simulink model "sampleModel2120_pp_difftest"  (R2021a)
settings: Solver=VariableStepAuto  StartTime=0.0  StopTime=10.0  RelTol=1e-3
undefined symbols (not defined in the file or in its folder): DiscIntNeverNeededParam, magnitude, Newton, Raphson
libraries: simulink x67, pid_lib x12
(part 1 of 3)
settings Model: Creator=lenovo  LastModifiedBy=user

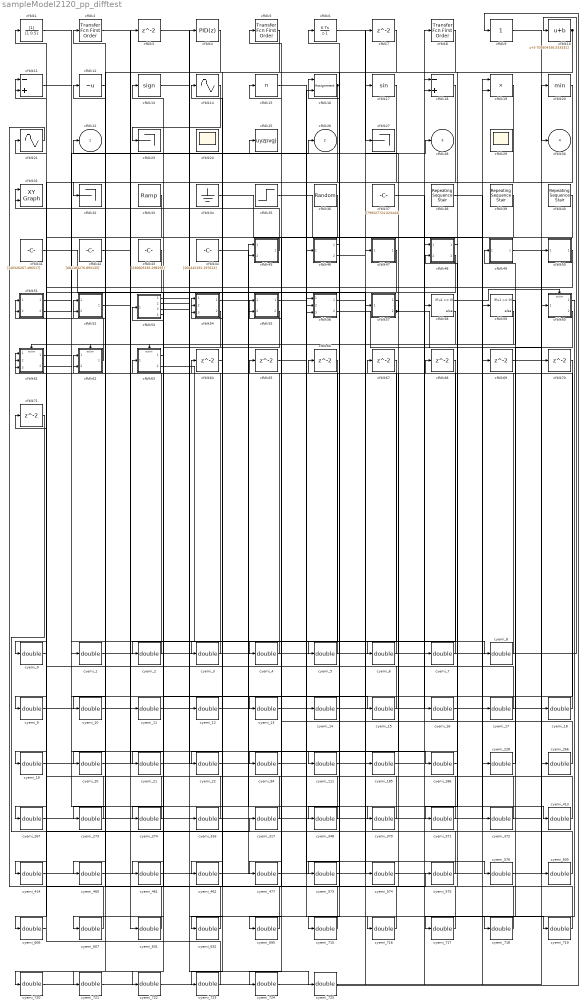
== system sampleModel2120_pp_difftest ==
  cfblk1 : DiscreteFilter  SampleTime=1
  cfblk10 : Bias  Bias=[-709504336.533331]
  cfblk11 : Sum  Inputs=-+  OutDataTypeStr=double
  cfblk12 : UnaryMinus
  cfblk13 : Signum
  cfblk14 : Sin  TimeSource=Use external signal  SampleTime=0
  cfblk15 : Product  Inputs=*  OutDataTypeStr=double
  cfblk16 : Assignment  DiagnosticForDimensions=Warning  IndexOptions=Index vector (dialog)  Indices=1  OutputSizes=1
  cfblk17 : Trigonometry
  cfblk18 : Sum  Inputs=-+  OutDataTypeStr=double
  cfblk19 : Product  Inputs=**  OutDataTypeStr=double
  cfblk2 : simulink/Discrete/Transfer Fcn First Order  PoleZ=0.95  ICPrevOutput=0.0  DoSatur=off
  cfblk20 : MinMax  OutDataTypeStr=double
  cfblk21 : Sin  TimeSource=Use external signal  SampleTime=0
  cfblk23 : Terminator
  cfblk24 : Scope
      settings: Floating=on
  cfblk25 : ToWorkspace  VariableName=uyzpvgj  SaveFormat=Timeseries  SampleTime=-1
  cfblk27 : Terminator
  cfblk29 : Scope
      settings: Floating=on
  cfblk{3,7,64..71} (10 alike) : Delay  SampleTime=1
  cfblk31 : simulink/Sinks/XY Graph  xmin=-1  xmax=1  ymin=-1  ymax=1  st=-1
  cfblk32 : Terminator
  cfblk33 : simulink/Sources/Ramp  slope=[-9170.423728]  start=[47.124759]  InitialOutput=[-914026.200250]
  cfblk34 : Ground
  cfblk35 : Step  Time=[9.000000]  Before=[-795213372.799819]  After=[478961987.281532]  SampleTime=0
  cfblk36 : RandomNumber  Mean=[10617.420643]  Variance=[21176.794349]  Seed=[230646429.000000]  SampleTime=0.1
  cfblk37 : Constant  Value=[799327724.023444]  OutDataTypeStr=double  SampleTime=1
  cfblk38 : simulink/Sources/Repeating Sequence Stair  OutValues=[-433408772.823916, -415254257.712957]  tsamp=1  OutMin=[]  OutMax=[]  OutDataTypeStr=double  OutputDataTypeScalingMode=double  OutDataType=fixdt(0,8)  ConRadixGroup=Best Precision: Vector-wise  OutScaling=2^-12
  cfblk39 : simulink/Sources/Repeating Sequence Stair  OutValues=[-289850517.751217, -807875800.203243]  tsamp=1  OutMin=[]  OutMax=[]  OutDataTypeStr=double  OutputDataTypeScalingMode=double  OutDataType=fixdt(0,8)  ConRadixGroup=Best Precision: Vector-wise  OutScaling=2^-12
  cfblk4 : pid_lib/PID Controller  Controller=PID  Form=Parallel  TimeDomain=Discrete-time  UseExternalTs=off  SampleTime=1  IntegratorMethod=Forward Euler  FilterMethod=Forward Euler  ControllerParametersSource=internal  P=1  I=1  D=0  UseFilter=on  N=100  TunerSelectOption=Transfer Function Based (PID Tuner App)  InitialConditionSource=internal  InitialConditionForIntegrator=0  InitialConditionForFilter=0  DifferentiatorICPrevScaledInput=0  ExternalReset=none  TrackingMode=off  Kt=1  LimitOutput=off  SatLimitsSource=internal  UpperSaturationLimit=inf  LowerSaturationLimit=-inf  LinearizeAsGain=off  AntiWindupMode=none  Kb=1  POutMin=[]  POutMax=[]  IOutMin=[]  IOutMax=[]  DOutMin=[]  DOutMax=[]  NOutMin=[]  NOutMax=[]  SumOutMin=[]  SumOutMax=[]  SaturationOutMin=[]  SaturationOutMax=[]  PParamMin=[]  PParamMax=[]  IParamMin=[]  IParamMax=[]  DParamMin=[]  DParamMax=[]  NParamMin=[]  NParamMax=[]  KbParamMin=[]  KbParamMax=[]  KtParamMin=[]  KtParamMax=[]  KbOutMin=[]  KbOutMax=[]  KtOutMin=[]  KtOutMax=[]  IntegratorOutMin=[]  IntegratorOutMax=[]  FilterOutMin=[]  FilterOutMax=[]  SumI1OutMin=[]  SumI1OutMax=[]  SumI2OutMin=[]  SumI2OutMax=[]  SumI3OutMin=[]  SumI3OutMax=[]  SumI4OutMin=[]  SumI4OutMax=[]  SumDOutMin=[]  SumDOutMax=[]  DifferentiatorOutMin=[]  DifferentiatorOutMax=[]  FilterDiffOutCoefMin=[]  FilterDiffOutCoefMax=[]  ReciprocalOutMin=[]  ReciprocalOutMax=[]  SumDenOutMin=[]  SumDenOutMax=[]  SumNumOutMin=[]  SumNumOutMax=[]  DivideOutMin=[]  DivideOutMax=[]  UdiffTsProdOutMin=[]  UdiffTsProdOutMax=[]  NTsProdOutMin=[]  NTsProdOutMax=[]  UintegralTsProdOutMin=[]  UintegralTsProdOutMax=[]  UngainTsProdOutMin=[]  UngainTsProdOutMax=[]  IntegratorContinuousStateAttributes=''  IntegratorStateMustResolveToSignalObject=off  IntegratorRTWStateStorageClass=Auto  FilterContinuousStateAttributes=''  FilterStateMustResolveToSignalObject=off  FilterRTWStateStorageClass=Auto  ParallelPVariant=InternalParameters  IdealPVariant=Disabled  IVariant=InternalParameters  DVariant=InternalParameters  IntegratorVariant=Discrete  SatVariant=Disabled  AWVariant=Passthrough  PCopyVariant=Disabled  TRVariant=Disabled  FdbkBlocksVariant=Forward  IdealPFdbkVariant=Disabled  SatFdbkVariant=Disabled  DerivativeFilterVariant=ForwardEulerFilter  NVariant=InternalParameters  NCopyVariant=Disabled  FilterICVariant=InternalICsFilter  IntegratorICVariant=InternalICs  ExternalResetVariant=Disabled  TRSumVariant=Passthrough  SumFdbkVariant=Disabled  SumVariant=Sum_PID  TsampFilterVariant=InternalTs  TsampNgainVariant=Passthrough  TsampIntegralVariant=Passthrough  ExternalSaturationOutDataTypeStr=Inherit: Same as second input
  cfblk40 : simulink/Sources/Repeating Sequence Stair  OutValues=[599228246.238422, -891664695.317547]  tsamp=1  OutMin=[]  OutMax=[]  OutDataTypeStr=double  OutputDataTypeScalingMode=double  OutDataType=fixdt(0,8)  ConRadixGroup=Best Precision: Vector-wise  OutScaling=2^-12
  cfblk41 : Constant  Value=[140326207.496517]  OutDataTypeStr=double  SampleTime=1
  cfblk42 : Constant  Value=[681184276.893135]  OutDataTypeStr=double  SampleTime=1
  cfblk43 : Constant  Value=[230605335.298195]  OutDataTypeStr=double  SampleTime=1
  cfblk44 : Constant  Value=[206442191.197613]  OutDataTypeStr=double  SampleTime=1
  cfblk45 : Subsystem
  cfblk46 : Subsystem
  cfblk47 : Subsystem
  cfblk48 : Subsystem
  cfblk49 : Subsystem
  cfblk5 : simulink/Discrete/Transfer Fcn First Order  PoleZ=0.95  ICPrevOutput=0.0  DoSatur=off
  cfblk50 : Subsystem
  cfblk51 : Subsystem
  cfblk52 : Subsystem
  cfblk53 : Subsystem
  cfblk54 : Subsystem
  cfblk55 : Subsystem
  cfblk56 : Subsystem
  cfblk57 : Subsystem
  cfblk58 : If  IfExpression=u1 >= 0  SampleTime=1
  cfblk59 : If  IfExpression=u1 >= 0  SampleTime=1
  cfblk6 : DiscreteIntegrator  OutDataTypeStr=double  ICPrevOutput=DiscIntNeverNeededParam  ICPrevScaledInput=DiscIntNeverNeededParam
  cfblk60 : Subsystem  TreatAsAtomicUnit=on
  cfblk61 : Subsystem  TreatAsAtomicUnit=on
  cfblk62 : Subsystem  TreatAsAtomicUnit=on
  cfblk63 : Subsystem  TreatAsAtomicUnit=on
  cfblk8 : simulink/Discrete/Transfer Fcn First Order  PoleZ=0.95  ICPrevOutput=0.0  DoSatur=off
  cfblk9 : simulink/Math Operations/Slider Gain  gain=1  low=0  high=2
  cyemi_{0..22,84,111,185..186,228,266..267,273..274,316..317,348,370..372,413..414,460..462,477,573..576,605..607,631..632,695,715..725} (65 alike) : DataTypeConversion  OutDataTypeStr=double
  cfblk22 : Outport
  cfblk26 : Outport  Port=2
  cfblk28 : Outport  Port=3
  cfblk30 : Outport  Port=4
  wires:
  cfblk45/1(cfblk2) -> cfblk31/1
  cfblk9/1 -> cfblk30/1
  cfblk14/1 -> cfblk23/1
  cfblk51/2(cfblk12) -> cfblk26/1
  cfblk57/2(cfblk17) -> cfblk22/1, cyemi_372/1
  cfblk46/2(cfblk8) -> cfblk28/1
  cfblk62/1(cfblk2) -> cfblk31/2
  cfblk16/1 -> cyemi_22/1, cyemi_723/1
  cfblk6/1 -> cfblk27/1
  cfblk4/1 -> cfblk32/1
  cfblk10/1 -> cyemi_3/1, cyemi_371/1
  cfblk58/1 -> cfblk60/Action
  cfblk58/2 -> cfblk61/Action
  cfblk59/1 -> cfblk62/Action
  cfblk59/2 -> cfblk63/Action
  cyemi_0/1 -> cfblk1/1
  cfblk33/1 -> cyemi_0/1
  cyemi_1/1 -> cfblk10/1
  cfblk61/2(cfblk14) -> cyemi_1/1
  cyemi_2/1 -> cfblk11/1
  cfblk66/1 -> cyemi_2/1
  cyemi_3/1 -> cfblk11/2
  cyemi_4/1 -> cfblk12/1
  cfblk63/2(cfblk8) -> cyemi_4/1
  cyemi_5/1 -> cfblk13/1
  cfblk54/1(cfblk2) -> cyemi_5/1
  cyemi_6/1 -> cfblk14/1
  cfblk1/1 -> cyemi_6/1
  cyemi_7/1 -> cfblk15/1
  cfblk37/1 -> cyemi_7/1
  cyemi_8/1 -> cfblk16/1
  cfblk52/1(cfblk2) -> cyemi_8/1
  cyemi_9/1 -> cfblk16/2
  cfblk17/1 -> cyemi_9/1
  cyemi_10/1 -> cfblk17/1
  cfblk12/1 -> cyemi_10/1
  cyemi_11/1 -> cfblk18/1
  cfblk2/1 -> cyemi_11/1
  cyemi_12/1 -> cfblk18/2
  cfblk53/3(cfblk6) -> cyemi_12/1
  cyemi_13/1 -> cfblk19/1
  cfblk61/1(cfblk2) -> cyemi_13/1
  cyemi_14/1 -> cfblk19/2
  cfblk15/1 -> cyemi_14/1
  cyemi_15/1 -> cfblk2/1
  cfblk53/1(cfblk2) -> cyemi_15/1
  cyemi_16/1 -> cfblk20/1
  cfblk34/1 -> cyemi_16/1
  cyemi_17/1 -> cfblk21/1
  cfblk35/1 -> cyemi_17/1
  cyemi_18/1 -> cfblk25/1
  cfblk56/2(cfblk12) -> cyemi_18/1
  cyemi_19/1 -> cfblk3/1
  cfblk50/1(cfblk2) -> cyemi_19/1
  cyemi_20/1 -> cfblk4/1
  cfblk47/1(cfblk2) -> cyemi_20/1
  cyemi_21/1 -> cfblk45/1(cfblk1)
  cfblk54/2(cfblk12) -> cyemi_21/1
  cyemi_22/1 -> cfblk45/2(cfblk15)
  cyemi_84/1 -> cfblk46/1(cfblk1)
  cfblk48/1(cfblk2) -> cyemi_84/1
  cyemi_111/1 -> cfblk47/1(cfblk1)
  cfblk57/1(cfblk2) -> cyemi_111/1
  cyemi_185/1 -> cfblk48/1(cfblk1)
  cfblk41/1 -> cyemi_185/1
  cyemi_186/1 -> cfblk48/2(cfblk13)
  cfblk11/1 -> cyemi_186/1
  cyemi_228/1 -> cfblk49/1(cfblk1)
  cfblk38/1 -> cyemi_228/1
  cyemi_266/1 -> cfblk5/1
  cfblk69/1 -> cyemi_266/1
  cyemi_267/1 -> cfblk50/1(cfblk1)
  cfblk18/1 -> cyemi_267/1
  cyemi_273/1 -> cfblk51/1(cfblk1)
  cfblk8/1 -> cyemi_273/1
  cyemi_274/1 -> cfblk51/2(cfblk11)
  cfblk53/4(cfblk7) -> cyemi_274/1
  cyemi_316/1 -> cfblk52/1(cfblk1)
  cfblk13/1 -> cyemi_316/1
  cyemi_317/1 -> cfblk52/2(cfblk15)
  cfblk71/1 -> cyemi_317/1
  cyemi_348/1 -> cfblk53/1(cfblk1)
  cfblk46/1(cfblk2) -> cyemi_348/1
  cyemi_370/1 -> cfblk54/1(cfblk1)
  cfblk44/1 -> cyemi_370/1
  cyemi_371/1 -> cfblk54/2(cfblk10)
  cyemi_372/1 -> cfblk54/3(cfblk11)
  cyemi_413/1 -> cfblk55/1(cfblk1)
  cfblk51/1(cfblk2) -> cyemi_413/1
  cyemi_414/1 -> cfblk55/2(cfblk10)
  cfblk20/1 -> cyemi_414/1
  cyemi_460/1 -> cfblk56/1(cfblk1)
  cfblk5/1 -> cyemi_460/1
  cyemi_461/1 -> cfblk56/2(cfblk10)
  cfblk70/1 -> cyemi_461/1
  cyemi_462/1 -> cfblk56/3(cfblk11)
  cfblk64/1 -> cyemi_462/1
  cyemi_477/1 -> cfblk57/1(cfblk1)
  cfblk39/1 -> cyemi_477/1
  cyemi_573/1 -> cfblk58/1
  cfblk7/1 -> cyemi_573/1
  cyemi_574/1 -> cfblk59/1
  cfblk56/1(cfblk2) -> cyemi_574/1
  cyemi_575/1 -> cfblk6/1
  cfblk21/1 -> cyemi_575/1
  cyemi_576/1 -> cfblk60/1(cfblk1)
  cfblk65/1 -> cyemi_576/1
  cyemi_605/1 -> cfblk61/1(cfblk1)
  cfblk49/1(cfblk2) -> cyemi_605/1
  cyemi_606/1 -> cfblk61/2(cfblk12)
  cfblk43/1 -> cyemi_606/1
  cyemi_607/1 -> cfblk61/3(cfblk13)
  cfblk63/1(cfblk2) -> cyemi_607/1
  cyemi_631/1 -> cfblk62/1(cfblk1)
  cfblk42/1 -> cyemi_631/1
  cyemi_632/1 -> cfblk62/2(cfblk13)
  cfblk67/1 -> cyemi_632/1
  cyemi_695/1 -> cfblk63/1(cfblk1)
  cfblk68/1 -> cyemi_695/1
  cyemi_715/1 -> cfblk64/1
  cfblk19/1 -> cyemi_715/1
  cyemi_716/1 -> cfblk65/1
  cfblk53/2(cfblk5) -> cyemi_716/1
  cyemi_717/1 -> cfblk66/1
  cfblk60/1(cfblk2) -> cyemi_717/1
  cyemi_718/1 -> cfblk67/1
  cfblk60/2(cfblk14) -> cyemi_718/1
  cyemi_719/1 -> cfblk68/1
  cfblk55/1(cfblk2) -> cyemi_719/1
  cyemi_720/1 -> cfblk69/1
  cfblk55/2(cfblk11) -> cyemi_720/1
  cyemi_721/1 -> cfblk7/1
  cfblk40/1 -> cyemi_721/1
  cyemi_722/1 -> cfblk70/1
  cfblk48/2(cfblk14) -> cyemi_722/1
  cyemi_723/1 -> cfblk71/1
  cyemi_724/1 -> cfblk8/1
  cfblk36/1 -> cyemi_724/1
  cyemi_725/1 -> cfblk9/1
  cfblk3/1 -> cyemi_725/1

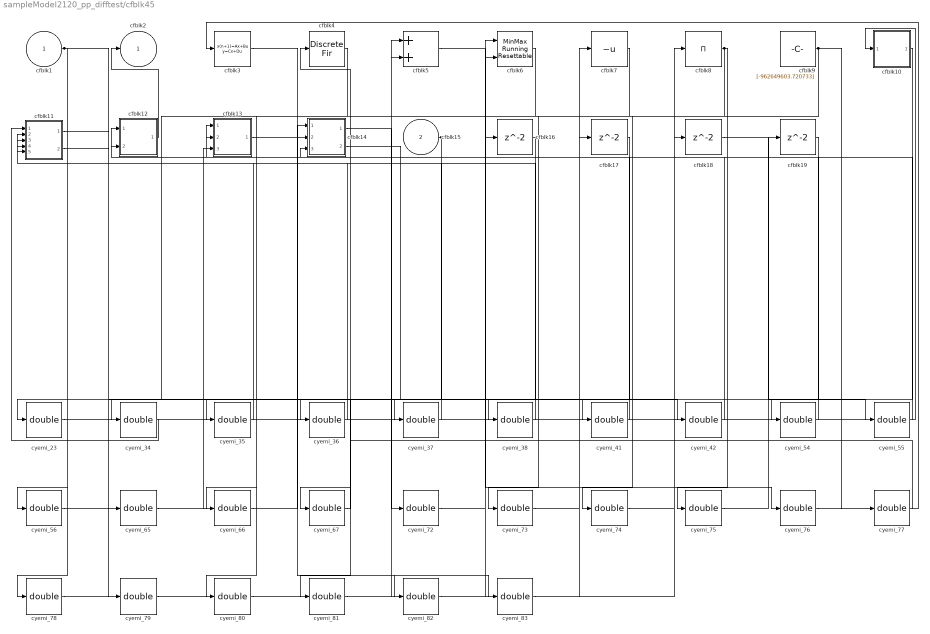
== system sampleModel2120_pp_difftest/cfblk45 ==
  cfblk1 : Inport
  cfblk15 : Inport  Port=2
  cfblk10 : Subsystem
  cfblk11 : Subsystem
  cfblk12 : Subsystem
  cfblk13 : Subsystem
  cfblk14 : Subsystem
  cfblk{16..19} (4 alike) : Delay  SampleTime=1
  cfblk3 : DiscreteStateSpace
  cfblk4 : DiscreteFir  SampleTime=1
  cfblk5 : Sum  OutDataTypeStr=double
  cfblk6 : simulink/Math Operations/MinMax Running Resettable  Function=min  vinit=0.0
  cfblk7 : UnaryMinus
  cfblk8 : Product  Inputs=*  OutDataTypeStr=double
  cfblk9 : Constant  Value=[-962649603.720733]  OutDataTypeStr=double  SampleTime=1
  cyemi_{23,34..38,41..42,54..56,65..67,72..83} (26 alike) : DataTypeConversion  OutDataTypeStr=double
  cfblk2 : Outport
  wires:
  cfblk12/1(cfblk2) -> cfblk2/1
  cfblk1/1 -> cyemi_23/1, cyemi_36/1, cyemi_42/1, cyemi_56/1
  cfblk9/1 -> cyemi_38/1, cyemi_77/1
  cfblk8/1 -> cyemi_73/1, cyemi_74/1, cyemi_75/1
  cyemi_23/1 -> cfblk10/1(cfblk1)
  cyemi_34/1 -> cfblk11/1(cfblk1)
  cfblk4/1 -> cyemi_34/1
  cyemi_35/1 -> cfblk11/2(cfblk6)
  cfblk6/1 -> cyemi_35/1
  cyemi_36/1 -> cfblk11/3(cfblk7)
  cyemi_37/1 -> cfblk11/4(cfblk8)
  cfblk19/1 -> cyemi_37/1
  cyemi_38/1 -> cfblk11/5(cfblk9)
  cyemi_41/1 -> cfblk12/1(cfblk1)
  cfblk14/2(cfblk9) -> cyemi_41/1
  cyemi_42/1 -> cfblk12/2(cfblk11)
  cyemi_54/1 -> cfblk13/1(cfblk1)
  cfblk10/1(cfblk2) -> cyemi_54/1
  cyemi_55/1 -> cfblk13/2(cfblk11)
  cfblk18/1 -> cyemi_55/1
  cyemi_56/1 -> cfblk13/3(cfblk12)
  cyemi_65/1 -> cfblk14/1(cfblk1)
  cfblk11/1(cfblk2) -> cyemi_65/1
  cyemi_66/1 -> cfblk14/2(cfblk7)
  cfblk15/1 -> cyemi_66/1, cyemi_67/1
  cyemi_67/1 -> cfblk14/3(cfblk8)
  cyemi_72/1 -> cfblk16/1
  cfblk14/1(cfblk2) -> cyemi_72/1
  cyemi_73/1 -> cfblk17/1
  cyemi_74/1 -> cfblk18/1
  cyemi_75/1 -> cfblk19/1
  cyemi_76/1 -> cfblk3/1
  cfblk5/1 -> cyemi_76/1
  cyemi_77/1 -> cfblk4/1
  cyemi_78/1 -> cfblk5/1
  cfblk17/1 -> cyemi_78/1
  cyemi_79/1 -> cfblk5/2
  cfblk11/2(cfblk10) -> cyemi_79/1
  cyemi_80/1 -> cfblk6/1
  cfblk7/1 -> cyemi_80/1
  cyemi_81/1 -> cfblk6/2
  cfblk16/1 -> cyemi_81/1
  cyemi_82/1 -> cfblk7/1
  cfblk13/1(cfblk2) -> cyemi_82/1
  cyemi_83/1 -> cfblk8/1
  cfblk3/1 -> cyemi_83/1

== system sampleModel2120_pp_difftest/cfblk46 ==
  cfblk1 : Inport
  cfblk10 : Delay  SampleTime=1
  cfblk11 : Delay  SampleTime=1
  cfblk3 : Signum
  cfblk4 : PermuteDimensions
  cfblk5 : simulink/Math Operations/MinMax Running Resettable  Function=min  vinit=0.0
  cfblk6 : Reshape
  cfblk7 : Subsystem
  cfblk9 : Delay  SampleTime=1
  cyemi_{85..95,110} (12 alike) : DataTypeConversion  OutDataTypeStr=double
  cfblk2 : Outport
  cfblk8 : Outport  Port=2
  wires:
  cfblk5/1 -> cfblk8/1, cyemi_85/1
  cfblk3/1 -> cfblk2/1, cyemi_86/1, cyemi_90/1
  cfblk7/2(cfblk17) -> cyemi_87/1, cyemi_91/1
  cyemi_85/1 -> cfblk10/1
  cyemi_86/1 -> cfblk11/1
  cyemi_87/1 -> cfblk3/1
  cyemi_88/1 -> cfblk4/1
  cfblk7/1(cfblk2) -> cyemi_88/1
  cyemi_89/1 -> cfblk5/1
  cfblk6/1 -> cyemi_89/1
  cyemi_90/1 -> cfblk5/2
  cyemi_91/1 -> cfblk6/1
  cyemi_92/1 -> cfblk7/1(cfblk1)
  cfblk9/1 -> cyemi_92/1
  cyemi_93/1 -> cfblk7/2(cfblk14)
  cfblk10/1 -> cyemi_93/1
  cyemi_94/1 -> cfblk7/3(cfblk15)
  cfblk11/1 -> cyemi_94/1
  cyemi_95/1 -> cfblk7/4(cfblk16)
  cfblk1/1 -> cyemi_95/1
  cyemi_110/1 -> cfblk9/1
  cfblk4/1 -> cyemi_110/1

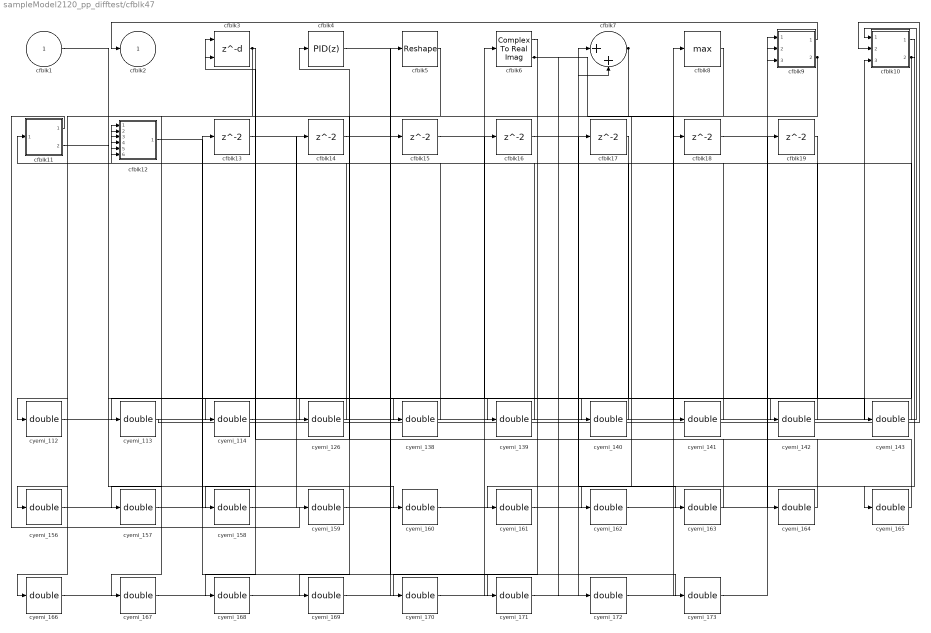
== system sampleModel2120_pp_difftest/cfblk47 ==
  cfblk1 : Inport
  cfblk10 : Subsystem
  cfblk11 : Subsystem
  cfblk12 : Subsystem
  cfblk{13..19} (7 alike) : Delay  SampleTime=1
  cfblk3 : Delay  DelayLengthSource=Input port  SampleTime=1
      settings: InputPortMap=u0,p1
  cfblk4 : pid_lib/PID Controller  Controller=PID  Form=Parallel  TimeDomain=Discrete-time  UseExternalTs=off  SampleTime=1  IntegratorMethod=Forward Euler  FilterMethod=Forward Euler  ControllerParametersSource=internal  P=1  I=1  D=0  UseFilter=on  N=100  TunerSelectOption=Transfer Function Based (PID Tuner App)  InitialConditionSource=internal  InitialConditionForIntegrator=0  InitialConditionForFilter=0  DifferentiatorICPrevScaledInput=0  ExternalReset=none  TrackingMode=off  Kt=1  LimitOutput=off  SatLimitsSource=internal  UpperSaturationLimit=inf  LowerSaturationLimit=-inf  LinearizeAsGain=off  AntiWindupMode=none  Kb=1  POutMin=[]  POutMax=[]  IOutMin=[]  IOutMax=[]  DOutMin=[]  DOutMax=[]  NOutMin=[]  NOutMax=[]  SumOutMin=[]  SumOutMax=[]  SaturationOutMin=[]  SaturationOutMax=[]  PParamMin=[]  PParamMax=[]  IParamMin=[]  IParamMax=[]  DParamMin=[]  DParamMax=[]  NParamMin=[]  NParamMax=[]  KbParamMin=[]  KbParamMax=[]  KtParamMin=[]  KtParamMax=[]  KbOutMin=[]  KbOutMax=[]  KtOutMin=[]  KtOutMax=[]  IntegratorOutMin=[]  IntegratorOutMax=[]  FilterOutMin=[]  FilterOutMax=[]  SumI1OutMin=[]  SumI1OutMax=[]  SumI2OutMin=[]  SumI2OutMax=[]  SumI3OutMin=[]  SumI3OutMax=[]  SumI4OutMin=[]  SumI4OutMax=[]  SumDOutMin=[]  SumDOutMax=[]  DifferentiatorOutMin=[]  DifferentiatorOutMax=[]  FilterDiffOutCoefMin=[]  FilterDiffOutCoefMax=[]  ReciprocalOutMin=[]  ReciprocalOutMax=[]  SumDenOutMin=[]  SumDenOutMax=[]  SumNumOutMin=[]  SumNumOutMax=[]  DivideOutMin=[]  DivideOutMax=[]  UdiffTsProdOutMin=[]  UdiffTsProdOutMax=[]  NTsProdOutMin=[]  NTsProdOutMax=[]  UintegralTsProdOutMin=[]  UintegralTsProdOutMax=[]  UngainTsProdOutMin=[]  UngainTsProdOutMax=[]  IntegratorContinuousStateAttributes=''  IntegratorStateMustResolveToSignalObject=off  IntegratorRTWStateStorageClass=Auto  FilterContinuousStateAttributes=''  FilterStateMustResolveToSignalObject=off  FilterRTWStateStorageClass=Auto  ParallelPVariant=InternalParameters  IdealPVariant=Disabled  IVariant=InternalParameters  DVariant=InternalParameters  IntegratorVariant=Discrete  SatVariant=Disabled  AWVariant=Passthrough  PCopyVariant=Disabled  TRVariant=Disabled  FdbkBlocksVariant=Forward  IdealPFdbkVariant=Disabled  SatFdbkVariant=Disabled  DerivativeFilterVariant=ForwardEulerFilter  NVariant=InternalParameters  NCopyVariant=Disabled  FilterICVariant=InternalICsFilter  IntegratorICVariant=InternalICs  ExternalResetVariant=Disabled  TRSumVariant=Passthrough  SumFdbkVariant=Disabled  SumVariant=Sum_PID  TsampFilterVariant=InternalTs  TsampNgainVariant=Passthrough  TsampIntegralVariant=Passthrough  ExternalSaturationOutDataTypeStr=Inherit: Same as second input
  cfblk5 : Reshape
  cfblk6 : ComplexToRealImag
  cfblk7 : Sum  Inputs=|++  OutDataTypeStr=double
  cfblk8 : MinMax  Function=max  OutDataTypeStr=double
  cfblk9 : Subsystem
  cyemi_{112..114,126,138..143,156..173} (28 alike) : DataTypeConversion  OutDataTypeStr=double
  cfblk2 : Outport
  wires:
  cfblk3/1 -> cyemi_113/1, cyemi_114/1, cyemi_168/1
  cfblk9/1(cfblk2) -> cfblk2/1
  cfblk10/2(cfblk15) -> cyemi_142/1, cyemi_165/1
  cfblk7/1 -> cyemi_112/1, cyemi_166/1
  cfblk6/2 -> cyemi_141/1, cyemi_172/1
  cfblk9/2(cfblk14) -> cyemi_156/1, cyemi_157/1, cyemi_158/1
  cyemi_112/1 -> cfblk10/1(cfblk1)
  cyemi_113/1 -> cfblk10/2(cfblk13)
  cyemi_114/1 -> cfblk10/3(cfblk14)
  cyemi_126/1 -> cfblk11/1(cfblk1)
  cfblk5/1 -> cyemi_126/1
  cyemi_138/1 -> cfblk12/1(cfblk1)
  cfblk1/1 -> cyemi_138/1
  cyemi_139/1 -> cfblk12/2(cfblk11)
  cfblk13/1 -> cyemi_139/1
  cyemi_140/1 -> cfblk12/3(cfblk12)
  cfblk14/1 -> cyemi_140/1
  cyemi_141/1 -> cfblk12/4(cfblk13)
  cyemi_142/1 -> cfblk12/5(cfblk14)
  cyemi_143/1 -> cfblk12/6(cfblk15)
  cfblk15/1 -> cyemi_143/1
  cyemi_156/1 -> cfblk13/1
  cyemi_157/1 -> cfblk14/1
  cyemi_158/1 -> cfblk15/1
  cyemi_159/1 -> cfblk16/1
  cfblk11/1(cfblk2) -> cyemi_159/1
  cyemi_160/1 -> cfblk17/1
  cfblk11/2(cfblk10) -> cyemi_160/1
  cyemi_161/1 -> cfblk18/1
  cfblk10/1(cfblk2) -> cyemi_161/1
  cyemi_162/1 -> cfblk19/1
  cfblk8/1 -> cyemi_162/1
  cyemi_163/1 -> cfblk3/1
  cfblk16/1 -> cyemi_163/1
  cyemi_164/1 -> cfblk3/2
  cfblk18/1 -> cyemi_164/1
  cyemi_165/1 -> cfblk4/1
  cyemi_166/1 -> cfblk5/1
  cyemi_167/1 -> cfblk6/1
  cfblk19/1 -> cyemi_167/1
  cyemi_168/1 -> cfblk7/1
  cyemi_169/1 -> cfblk7/2
  cfblk17/1 -> cyemi_169/1
  cyemi_170/1 -> cfblk8/1
  cfblk6/1 -> cyemi_170/1
  cyemi_171/1 -> cfblk9/1(cfblk1)
  cfblk4/1 -> cyemi_171/1
  cyemi_172/1 -> cfblk9/2(cfblk12)
  cyemi_173/1 -> cfblk9/3(cfblk13)
  cfblk12/1(cfblk2) -> cyemi_173/1

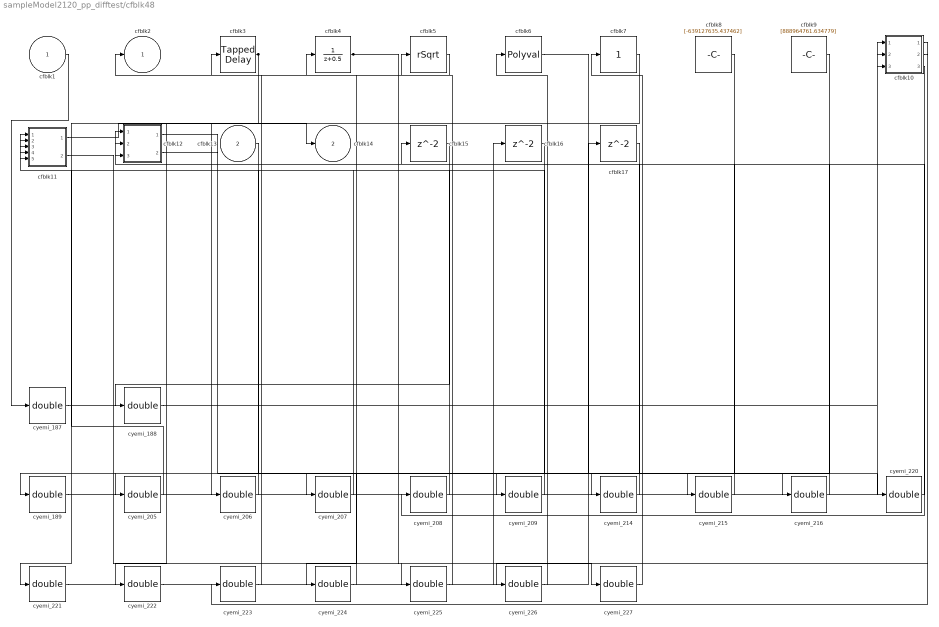
== system sampleModel2120_pp_difftest/cfblk48 ==
  cfblk1 : Inport
  cfblk13 : Inport  Port=2
  cfblk10 : Subsystem
  cfblk11 : Subsystem
  cfblk12 : Subsystem
  cfblk15 : Delay  SampleTime=1
  cfblk16 : Delay  SampleTime=1
  cfblk17 : Delay  SampleTime=1
  cfblk3 : simulink/Discrete/Tapped Delay  vinit=0.0  samptime=-1  NumDelays=1  DelayOrder=Oldest  includeCurrent=off
  cfblk4 : DiscreteTransferFcn  SampleTime=1
  cfblk5 : Sqrt  Operator=rSqrt  OutDataTypeStr=double  AlgorithmType=Newton-Raphson  SaturateOnIntegerOverflow=on
  cfblk6 : Polyval  Coefs=[ +2.081618890e-019, -1.441693666e-014, +4.719686976e-010, -8.536869453e-006, +1.621573104e-001, -8.087801117e+001 ]
  cfblk7 : simulink/Math Operations/Slider Gain  gain=1  low=0  high=2
  cfblk8 : Constant  Value=[-639127635.437462]  OutDataTypeStr=double  SampleTime=1
  cfblk9 : Constant  Value=[888964761.634779]  OutDataTypeStr=double  SampleTime=1
  cyemi_{187..189,205..209,214..216,220..227} (19 alike) : DataTypeConversion  OutDataTypeStr=double
  cfblk2 : Outport
  cfblk14 : Outport  Port=2
  wires:
  cfblk4/1 -> cyemi_209/1, cyemi_227/1
  cfblk5/1 -> cfblk2/1
  cfblk11/1(cfblk2) -> cfblk14/1
  cfblk3/1 -> cyemi_206/1, cyemi_221/1
  cyemi_187/1 -> cfblk10/1(cfblk1)
  cfblk1/1 -> cyemi_187/1
  cyemi_188/1 -> cfblk10/2(cfblk14)
  cfblk15/1 -> cyemi_188/1
  cyemi_189/1 -> cfblk10/3(cfblk15)
  cfblk16/1 -> cyemi_189/1
  cyemi_205/1 -> cfblk11/1(cfblk1)
  cfblk13/1 -> cyemi_205/1
  cyemi_206/1 -> cfblk11/2(cfblk7)
  cyemi_207/1 -> cfblk11/3(cfblk8)
  cfblk12/2(cfblk10) -> cyemi_207/1
  cyemi_208/1 -> cfblk11/4(cfblk9)
  cfblk10/3(cfblk17) -> cyemi_208/1
  cyemi_209/1 -> cfblk11/5(cfblk10)
  cyemi_214/1 -> cfblk12/1(cfblk1)
  cfblk9/1 -> cyemi_214/1
  cyemi_215/1 -> cfblk12/2(cfblk8)
  cfblk8/1 -> cyemi_215/1
  cyemi_216/1 -> cfblk12/3(cfblk9)
  cfblk6/1 -> cyemi_216/1
  cyemi_220/1 -> cfblk15/1
  cfblk12/1(cfblk2) -> cyemi_220/1
  cyemi_221/1 -> cfblk16/1
  cyemi_222/1 -> cfblk17/1
  cfblk7/1 -> cyemi_222/1
  cyemi_223/1 -> cfblk3/1
  cfblk10/2(cfblk16) -> cyemi_223/1
  cyemi_224/1 -> cfblk4/1
  cfblk17/1 -> cyemi_224/1
  cyemi_225/1 -> cfblk5/1
  cfblk11/2(cfblk11) -> cyemi_225/1
  cyemi_226/1 -> cfblk6/1
  cfblk10/1(cfblk2) -> cyemi_226/1
  cyemi_227/1 -> cfblk7/1

== system sampleModel2120_pp_difftest/cfblk49 ==
  cfblk1 : Inport
  cfblk{8..12} (5 alike) : Delay  SampleTime=1
  cfblk3 : Polyval  Coefs=[ +2.081618890e-019, -1.441693666e-014, +4.719686976e-010, -8.536869453e-006, +1.621573104e-001, -8.087801117e+001 ]
  cfblk4 : Reshape
  cfblk5 : Subsystem
  cfblk6 : Subsystem
  cfblk7 : Subsystem
  cyemi_{229..235,241..245,253..255,264..265} (17 alike) : DataTypeConversion  OutDataTypeStr=double
  cfblk2 : Outport
  wires:
  cfblk3/1 -> cyemi_229/1, cyemi_233/1
  cfblk4/1 -> cyemi_264/1, cyemi_265/1
  cfblk5/1(cfblk2) -> cfblk2/1, cyemi_230/1, cyemi_231/1
  cyemi_229/1 -> cfblk10/1
  cyemi_230/1 -> cfblk11/1
  cyemi_231/1 -> cfblk12/1
  cyemi_232/1 -> cfblk3/1
  cfblk6/1(cfblk2) -> cyemi_232/1
  cyemi_233/1 -> cfblk4/1
  cyemi_234/1 -> cfblk5/1(cfblk1)
  cfblk7/1(cfblk2) -> cyemi_234/1
  cyemi_235/1 -> cfblk5/2(cfblk7)
  cfblk6/3(cfblk16) -> cyemi_235/1
  cyemi_241/1 -> cfblk6/1(cfblk1)
  cfblk8/1 -> cyemi_241/1
  cyemi_242/1 -> cfblk6/2(cfblk11)
  cfblk1/1 -> cyemi_242/1
  cyemi_243/1 -> cfblk6/3(cfblk12)
  cfblk10/1 -> cyemi_243/1
  cyemi_244/1 -> cfblk6/4(cfblk13)
  cfblk11/1 -> cyemi_244/1
  cyemi_245/1 -> cfblk6/5(cfblk14)
  cfblk9/1 -> cyemi_245/1
  cyemi_253/1 -> cfblk7/1(cfblk1)
  cfblk6/2(cfblk15) -> cyemi_253/1
  cyemi_254/1 -> cfblk7/2(cfblk12)
  cfblk6/4(cfblk17) -> cyemi_254/1
  cyemi_255/1 -> cfblk7/3(cfblk13)
  cfblk12/1 -> cyemi_255/1
  cyemi_264/1 -> cfblk8/1
  cyemi_265/1 -> cfblk9/1

== system sampleModel2120_pp_difftest/cfblk50 ==
  cfblk1 : Inport
  cfblk3 : simulink/Discrete/Difference  ICPrevInput=0.0  OutMin=[]  OutMax=[]  OutDataTypeStr=double  OutputDataTypeScalingMode=double  OutDataType=fixdt(1, 16)  OutScaling=2^-10  DoSatur=off
  cfblk4 : simulink/Discrete/Transfer Fcn Real Zero  ZeroZ=0.75  ICPrevInput=0.0  DoSatur=off
      settings: SourceProductBaseCode=SL
  cfblk5 : simulink/Discrete/Transfer Fcn First Order  PoleZ=0.95  ICPrevOutput=0.0  DoSatur=off
  cfblk6 : simulink/Discrete/Difference  ICPrevInput=0.0  OutMin=[]  OutMax=[]  OutDataTypeStr=double  OutputDataTypeScalingMode=double  OutDataType=fixdt(1, 16)  OutScaling=2^-10  DoSatur=off
  cfblk7 : Sin  TimeSource=Use external signal  SampleTime=0
  cyemi_{268..272} (5 alike) : DataTypeConversion  OutDataTypeStr=double
  cfblk2 : Outport
  wires:
  cfblk6/1 -> cfblk2/1
  cyemi_268/1 -> cfblk3/1
  cfblk5/1 -> cyemi_268/1
  cyemi_269/1 -> cfblk4/1
  cfblk7/1 -> cyemi_269/1
  cyemi_270/1 -> cfblk5/1
  cfblk1/1 -> cyemi_270/1
  cyemi_271/1 -> cfblk6/1
  cfblk4/1 -> cyemi_271/1
  cyemi_272/1 -> cfblk7/1
  cfblk3/1 -> cyemi_272/1

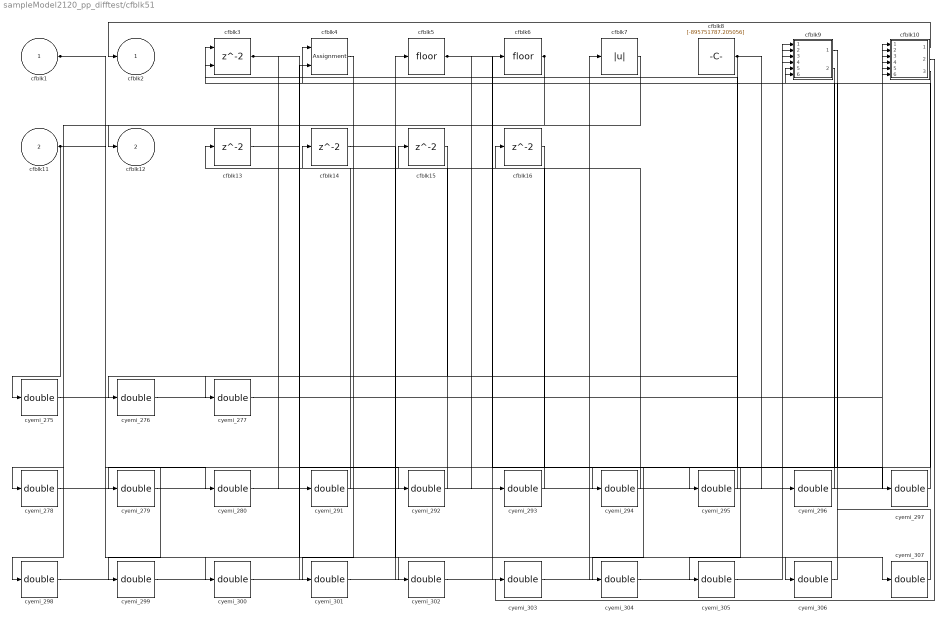
== system sampleModel2120_pp_difftest/cfblk51 ==
  cfblk1 : Inport
  cfblk11 : Inport  Port=2
  cfblk10 : Subsystem
  cfblk{13..16} (4 alike) : Delay  SampleTime=1
  cfblk3 : Delay  ShowEnablePort=on  SampleTime=1
      settings: InputPortMap=u0,e6
  cfblk4 : Assignment  DiagnosticForDimensions=Warning  IndexOptions=Index vector (dialog)  Indices=1  OutputSizes=1
  cfblk5 : Rounding
  cfblk6 : Rounding
  cfblk7 : Abs  OutDataTypeStr=double
  cfblk8 : Constant  Value=[-895751787.205056]  OutDataTypeStr=double  SampleTime=1
  cfblk9 : Subsystem
  cyemi_{275..280,291..307} (23 alike) : DataTypeConversion  OutDataTypeStr=double
  cfblk2 : Outport
  cfblk12 : Outport  Port=2
  wires:
  cfblk5/1 -> cyemi_293/1, cyemi_294/1, cyemi_297/1
  cfblk7/1 -> cfblk12/1
  cfblk11/1 -> cyemi_275/1, cyemi_306/1
  cfblk1/1 -> cyemi_280/1, cyemi_300/1
  cfblk6/1 -> cyemi_278/1, cyemi_298/1
  cfblk10/1(cfblk2) -> cfblk2/1
  cfblk3/1 -> cyemi_291/1, cyemi_292/1
  cfblk8/1 -> cyemi_277/1, cyemi_296/1, cyemi_304/1
  cyemi_275/1 -> cfblk10/1(cfblk1)
  cyemi_276/1 -> cfblk10/2(cfblk11)
  cfblk15/1 -> cyemi_276/1
  cyemi_277/1 -> cfblk10/3(cfblk12)
  cyemi_278/1 -> cfblk10/4(cfblk13)
  cyemi_279/1 -> cfblk10/5(cfblk14)
  cfblk16/1 -> cyemi_279/1
  cyemi_280/1 -> cfblk10/6(cfblk15)
  cyemi_291/1 -> cfblk13/1
  cyemi_292/1 -> cfblk14/1
  cyemi_293/1 -> cfblk15/1
  cyemi_294/1 -> cfblk16/1
  cyemi_295/1 -> cfblk3/1
  cfblk9/1(cfblk2) -> cyemi_295/1
  cyemi_296/1 -> cfblk3/2
  cyemi_297/1 -> cfblk4/1
  cyemi_298/1 -> cfblk4/2
  cyemi_299/1 -> cfblk5/1
  cfblk9/2(cfblk14) -> cyemi_299/1
  cyemi_300/1 -> cfblk6/1
  cyemi_301/1 -> cfblk7/1
  cfblk4/1 -> cyemi_301/1
  cyemi_302/1 -> cfblk9/1(cfblk1)
  cfblk13/1 -> cyemi_302/1
  cyemi_303/1 -> cfblk9/2(cfblk9)
  cfblk10/2(cfblk16) -> cyemi_303/1
  cyemi_304/1 -> cfblk9/3(cfblk10)
  cyemi_305/1 -> cfblk9/4(cfblk11)
  cfblk10/3(cfblk17) -> cyemi_305/1
  cyemi_306/1 -> cfblk9/5(cfblk12)
  cyemi_307/1 -> cfblk9/6(cfblk13)
  cfblk14/1 -> cyemi_307/1

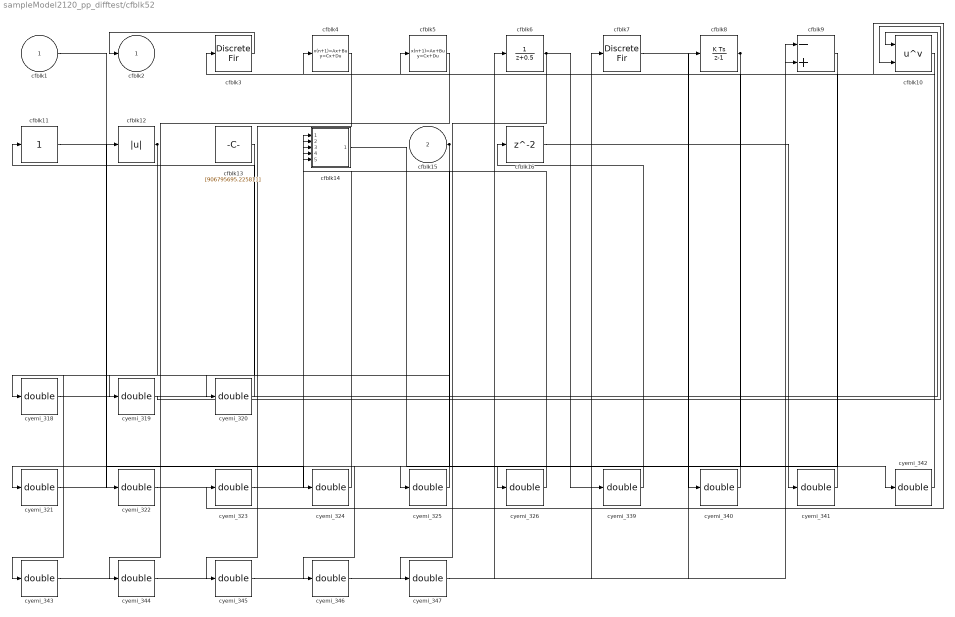
== system sampleModel2120_pp_difftest/cfblk52 ==
  cfblk1 : Inport
  cfblk15 : Inport  Port=2
  cfblk10 : Math  Operator=pow  OutDataTypeStr=double  SaturateOnIntegerOverflow=on
  cfblk11 : simulink/Math Operations/Slider Gain  gain=1  low=0  high=2
  cfblk12 : Abs  OutDataTypeStr=double
  cfblk13 : Constant  Value=[906795695.225811]  OutDataTypeStr=double  SampleTime=1
  cfblk14 : Subsystem
  cfblk16 : Delay  SampleTime=1
  cfblk3 : DiscreteFir  SampleTime=1
  cfblk4 : DiscreteStateSpace
  cfblk5 : DiscreteStateSpace
  cfblk6 : DiscreteTransferFcn  SampleTime=1
  cfblk7 : DiscreteFir  SampleTime=1
  cfblk8 : DiscreteIntegrator  OutDataTypeStr=double  ICPrevOutput=DiscIntNeverNeededParam  ICPrevScaledInput=DiscIntNeverNeededParam
  cfblk9 : Sum  Inputs=-+  OutDataTypeStr=double
  cyemi_{318..326,339..347} (18 alike) : DataTypeConversion  OutDataTypeStr=double
  cfblk2 : Outport
  wires:
  cfblk12/1 -> cyemi_319/1, cyemi_343/1
  cfblk15/1 -> cyemi_318/1, cyemi_345/1
  cfblk3/1 -> cfblk2/1
  cfblk8/1 -> cyemi_326/1, cyemi_346/1
  cfblk6/1 -> cyemi_339/1, cyemi_347/1
  cyemi_318/1 -> cfblk10/1
  cyemi_319/1 -> cfblk10/2
  cyemi_320/1 -> cfblk11/1
  cfblk13/1 -> cyemi_320/1
  cyemi_321/1 -> cfblk12/1
  cfblk4/1 -> cyemi_321/1
  cyemi_322/1 -> cfblk14/1(cfblk1)
  cfblk1/1 -> cyemi_322/1
  cyemi_323/1 -> cfblk14/2(cfblk14)
  cfblk10/1 -> cyemi_323/1
  cyemi_324/1 -> cfblk14/3(cfblk15)
  cfblk11/1 -> cyemi_324/1
  cyemi_325/1 -> cfblk14/4(cfblk16)
  cfblk9/1 -> cyemi_325/1
  cyemi_326/1 -> cfblk14/5(cfblk17)
  cyemi_339/1 -> cfblk16/1
  cyemi_340/1 -> cfblk3/1
  cfblk7/1 -> cyemi_340/1
  cyemi_341/1 -> cfblk4/1
  cfblk16/1 -> cyemi_341/1
  cyemi_342/1 -> cfblk5/1
  cfblk14/1(cfblk2) -> cyemi_342/1
  cyemi_343/1 -> cfblk6/1
  cyemi_344/1 -> cfblk7/1
  cfblk5/1 -> cyemi_344/1
  cyemi_345/1 -> cfblk8/1
  cyemi_346/1 -> cfblk9/1
  cyemi_347/1 -> cfblk9/2

== system sampleModel2120_pp_difftest/cfblk53 ==
  cfblk1 : Inport
  cfblk3 : Subsystem
  cfblk4 : Subsystem
  cyemi_{349..350,360..362} (5 alike) : DataTypeConversion  OutDataTypeStr=double
  cfblk2 : Outport
  cfblk5 : Outport  Port=2
  cfblk6 : Outport  Port=3
  cfblk7 : Outport  Port=4
  wires:
  cfblk1/1 -> cfblk2/1, cyemi_349/1, cyemi_350/1
  cfblk3/1(cfblk2) -> cfblk5/1
  cfblk3/5(cfblk13) -> cfblk7/1
  cfblk4/1(cfblk2) -> cfblk6/1
  cyemi_349/1 -> cfblk3/1(cfblk1)
  cyemi_350/1 -> cfblk3/2(cfblk9)
  cyemi_360/1 -> cfblk4/1(cfblk1)
  cfblk3/2(cfblk10) -> cyemi_360/1
  cyemi_361/1 -> cfblk4/2(cfblk8)
  cfblk3/3(cfblk11) -> cyemi_361/1
  cyemi_362/1 -> cfblk4/3(cfblk9)
  cfblk3/4(cfblk12) -> cyemi_362/1

== system sampleModel2120_pp_difftest/cfblk54 ==
  cfblk1 : Inport
  cfblk10 : Inport  Port=2
  cfblk11 : Inport  Port=3
  cfblk13 : Delay  SampleTime=1
  cfblk3 : DiscreteFir  SampleTime=1
  cfblk4 : Math  Operator=magnitude^2  OutDataTypeStr=double  SaturateOnIntegerOverflow=on
  cfblk5 : PermuteDimensions
  cfblk6 : Subsystem
  cfblk7 : Subsystem
  cfblk8 : Subsystem
  cfblk9 : Subsystem
  cyemi_{373..381,387,396,408..409} (13 alike) : DataTypeConversion  OutDataTypeStr=double
  cfblk2 : Outport
  cfblk12 : Outport  Port=2
  wires:
  cfblk3/1 -> cfblk2/1
  cfblk9/2(cfblk8) -> cfblk12/1
  cfblk8/1(cfblk2) -> cyemi_376/1, cyemi_380/1, cyemi_381/1
  cyemi_373/1 -> cfblk13/1
  cfblk6/1(cfblk2) -> cyemi_373/1
  cyemi_374/1 -> cfblk3/1
  cfblk10/1 -> cyemi_374/1
  cyemi_375/1 -> cfblk4/1
  cfblk5/1 -> cyemi_375/1
  cyemi_376/1 -> cfblk5/1
  cyemi_377/1 -> cfblk6/1(cfblk1)
  cfblk7/1(cfblk2) -> cyemi_377/1
  cyemi_378/1 -> cfblk6/2(cfblk9)
  cfblk9/3(cfblk9) -> cyemi_378/1
  cyemi_379/1 -> cfblk6/3(cfblk10)
  cfblk4/1 -> cyemi_379/1
  cyemi_380/1 -> cfblk6/4(cfblk11)
  cyemi_381/1 -> cfblk6/5(cfblk12)
  cyemi_387/1 -> cfblk7/1(cfblk1)
  cfblk11/1 -> cyemi_387/1
  cyemi_396/1 -> cfblk8/1(cfblk1)
  cfblk9/1(cfblk2) -> cyemi_396/1
  cyemi_408/1 -> cfblk9/1(cfblk1)
  cfblk1/1 -> cyemi_408/1
  cyemi_409/1 -> cfblk9/2(cfblk7)
  cfblk13/1 -> cyemi_409/1

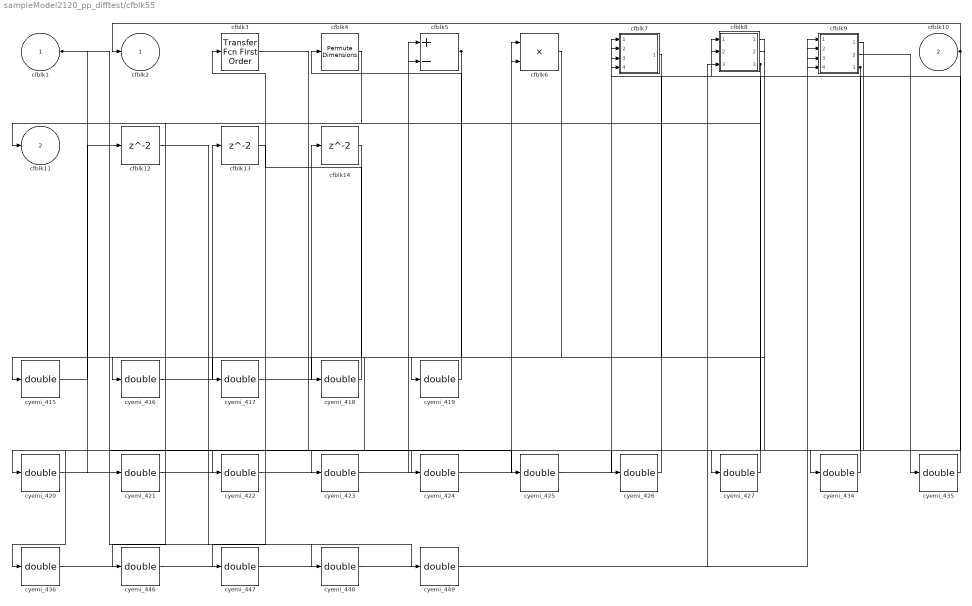
== system sampleModel2120_pp_difftest/cfblk55 ==
  cfblk1 : Inport
  cfblk10 : Inport  Port=2
  cfblk12 : Delay  SampleTime=1
  cfblk13 : Delay  SampleTime=1
  cfblk14 : Delay  SampleTime=1
  cfblk3 : simulink/Discrete/Transfer Fcn First Order  PoleZ=0.95  ICPrevOutput=0.0  DoSatur=off
  cfblk4 : PermuteDimensions
  cfblk5 : Sum  Inputs=+-  OutDataTypeStr=double
  cfblk6 : Product  Inputs=**  OutDataTypeStr=double
  cfblk7 : Subsystem
  cfblk8 : Subsystem
  cfblk9 : Subsystem
  cyemi_{415..427,434..436,446..449} (20 alike) : DataTypeConversion  OutDataTypeStr=double
  cfblk2 : Outport
  cfblk11 : Outport  Port=2
  wires:
  cfblk5/1 -> cyemi_418/1, cyemi_423/1
  cfblk10/1 -> cfblk2/1, cyemi_426/1
  cfblk1/1 -> cyemi_421/1, cyemi_425/1, cyemi_449/1
  cfblk9/3(cfblk16) -> cyemi_420/1, cyemi_436/1
  cfblk8/3(cfblk13) -> cfblk11/1, cyemi_427/1
  cyemi_415/1 -> cfblk12/1
  cfblk6/1 -> cyemi_415/1
  cyemi_416/1 -> cfblk13/1
  cfblk4/1 -> cyemi_416/1
  cyemi_417/1 -> cfblk14/1
  cfblk7/1(cfblk2) -> cyemi_417/1
  cyemi_418/1 -> cfblk3/1
  cyemi_419/1 -> cfblk4/1
  cfblk8/2(cfblk12) -> cyemi_419/1
  cyemi_420/1 -> cfblk5/1
  cyemi_421/1 -> cfblk5/2
  cyemi_422/1 -> cfblk6/1
  cfblk8/1(cfblk2) -> cyemi_422/1
  cyemi_423/1 -> cfblk6/2
  cyemi_424/1 -> cfblk7/1(cfblk1)
  cfblk3/1 -> cyemi_424/1
  cyemi_425/1 -> cfblk7/2(cfblk7)
  cyemi_426/1 -> cfblk7/3(cfblk8)
  cyemi_427/1 -> cfblk7/4(cfblk9)
  cyemi_434/1 -> cfblk8/1(cfblk1)
  cfblk9/1(cfblk2) -> cyemi_434/1
  cyemi_435/1 -> cfblk8/2(cfblk10)
  cfblk9/2(cfblk15) -> cyemi_435/1
  cyemi_436/1 -> cfblk8/3(cfblk11)
  cyemi_446/1 -> cfblk9/1(cfblk1)
  cfblk14/1 -> cyemi_446/1
  cyemi_447/1 -> cfblk9/2(cfblk12)
  cfblk13/1 -> cyemi_447/1
  cyemi_448/1 -> cfblk9/3(cfblk13)
  cfblk12/1 -> cyemi_448/1
  cyemi_449/1 -> cfblk9/4(cfblk14)

== system sampleModel2120_pp_difftest/cfblk56 ==
  cfblk1 : Inport
  cfblk10 : Inport  Port=2
  cfblk11 : Inport  Port=3
  cfblk3 : DiscreteFilter  SampleTime=1
  cfblk4 : UnitDelay  HasFrameUpgradeWarning=on
  cfblk5 : simulink/Discrete/Difference  ICPrevInput=0.0  OutMin=[]  OutMax=[]  OutDataTypeStr=double  OutputDataTypeScalingMode=double  OutDataType=fixdt(1, 16)  OutScaling=2^-10  DoSatur=off
  cfblk6 : PermuteDimensions
  cfblk7 : Reshape
  cfblk8 : Constant  Value=[483167932.969646]  OutDataTypeStr=double  SampleTime=1
  cfblk9 : Subsystem
  cyemi_{463..470} (8 alike) : DataTypeConversion  OutDataTypeStr=double
  cfblk2 : Outport
  cfblk12 : Outport  Port=2
  wires:
  cfblk3/1 -> cfblk2/1
  cfblk4/1 -> cfblk12/1
  cyemi_463/1 -> cfblk3/1
  cfblk5/1 -> cyemi_463/1
  cyemi_464/1 -> cfblk4/1
  cfblk6/1 -> cyemi_464/1
  cyemi_465/1 -> cfblk5/1
  cfblk7/1 -> cyemi_465/1
  cyemi_466/1 -> cfblk6/1
  cfblk10/1 -> cyemi_466/1
  cyemi_467/1 -> cfblk7/1
  cfblk9/1(cfblk2) -> cyemi_467/1
  cyemi_468/1 -> cfblk9/1(cfblk1)
  cfblk8/1 -> cyemi_468/1
  cyemi_469/1 -> cfblk9/2(cfblk8)
  cfblk11/1 -> cyemi_469/1
  cyemi_470/1 -> cfblk9/3(cfblk9)
  cfblk1/1 -> cyemi_470/1

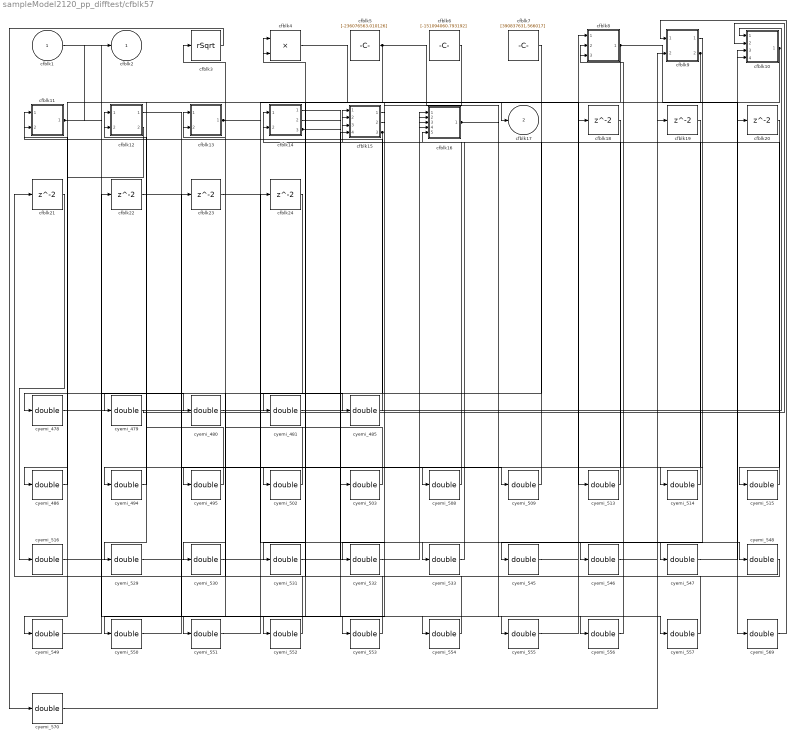
== system sampleModel2120_pp_difftest/cfblk57 ==
  cfblk1 : Inport
  cfblk10 : Subsystem
  cfblk11 : Subsystem
  cfblk12 : Subsystem
  cfblk13 : Subsystem
  cfblk14 : Subsystem
  cfblk15 : Subsystem
  cfblk16 : Subsystem
  cfblk{18..24} (7 alike) : Delay  SampleTime=1
  cfblk3 : Sqrt  Operator=rSqrt  OutDataTypeStr=double  AlgorithmType=Newton-Raphson  SaturateOnIntegerOverflow=on
  cfblk4 : Product  Inputs=**  OutDataTypeStr=double
  cfblk5 : Constant  Value=[-236076563.010126]  OutDataTypeStr=double  SampleTime=1
  cfblk6 : Constant  Value=[-151094060.793192]  OutDataTypeStr=double  SampleTime=1
  cfblk7 : Constant  Value=[390837631.566017]  OutDataTypeStr=double  SampleTime=1
  cfblk8 : Subsystem
  cfblk9 : Subsystem
  cyemi_{478..481,485..486,494..495,502..503,508..509,513..516,529..533,545..557,569..570} (36 alike) : DataTypeConversion  OutDataTypeStr=double
  cfblk2 : Outport
  cfblk17 : Outport  Port=2
  wires:
  cfblk16/1(cfblk2) -> cyemi_546/1, cyemi_547/1
  cfblk10/1(cfblk2) -> cyemi_486/1, cyemi_514/1
  cfblk13/1(cfblk2) -> cfblk17/1, cyemi_533/1
  cfblk8/1(cfblk2) -> cyemi_552/1, cyemi_569/1
  cfblk5/1 -> cyemi_502/1, cyemi_557/1
  cfblk11/1(cfblk2) -> cfblk2/1, cyemi_554/1
  cfblk15/3(cfblk17) -> cyemi_530/1, cyemi_551/1
  cfblk14/3(cfblk8) -> cyemi_548/1, cyemi_556/1
  cyemi_478/1 -> cfblk10/1(cfblk1)
  cfblk7/1 -> cyemi_478/1
  cyemi_479/1 -> cfblk10/2(cfblk6)
  cfblk6/1 -> cyemi_479/1
  cyemi_480/1 -> cfblk10/3(cfblk7)
  cfblk1/1 -> cyemi_480/1
  cyemi_481/1 -> cfblk10/4(cfblk8)
  cfblk24/1 -> cyemi_481/1
  cyemi_485/1 -> cfblk11/1(cfblk1)
  cfblk23/1 -> cyemi_485/1
  cyemi_486/1 -> cfblk11/2(cfblk9)
  cyemi_494/1 -> cfblk12/1(cfblk1)
  cfblk19/1 -> cyemi_494/1
  cyemi_495/1 -> cfblk12/2(cfblk8)
  cfblk15/1(cfblk2) -> cyemi_495/1
  cyemi_502/1 -> cfblk13/1(cfblk1)
  cyemi_503/1 -> cfblk13/2(cfblk7)
  cfblk14/2(cfblk7) -> cyemi_503/1
  cyemi_508/1 -> cfblk14/1(cfblk1)
  cfblk18/1 -> cyemi_508/1
  cyemi_509/1 -> cfblk14/2(cfblk6)
  cfblk12/1(cfblk2) -> cyemi_509/1
  cyemi_513/1 -> cfblk15/1(cfblk1)
  cfblk4/1 -> cyemi_513/1
  cyemi_514/1 -> cfblk15/2(cfblk13)
  cyemi_515/1 -> cfblk15/3(cfblk14)
  cfblk20/1 -> cyemi_515/1
  cyemi_516/1 -> cfblk15/4(cfblk15)
  cfblk21/1 -> cyemi_516/1
  cyemi_529/1 -> cfblk16/1(cfblk1)
  cfblk9/2(cfblk7) -> cyemi_529/1, cyemi_531/1, cyemi_532/1
  cyemi_530/1 -> cfblk16/2(cfblk13)
  cyemi_531/1 -> cfblk16/3(cfblk14)
  cyemi_532/1 -> cfblk16/4(cfblk15)
  cyemi_533/1 -> cfblk16/5(cfblk16)
  cyemi_545/1 -> cfblk18/1
  cfblk9/1(cfblk2) -> cyemi_545/1
  cyemi_546/1 -> cfblk19/1
  cyemi_547/1 -> cfblk20/1
  cyemi_548/1 -> cfblk21/1
  cyemi_549/1 -> cfblk22/1
  cfblk12/2(cfblk9) -> cyemi_549/1
  cyemi_550/1 -> cfblk23/1
  cfblk15/2(cfblk16) -> cyemi_550/1
  cyemi_551/1 -> cfblk24/1
  cyemi_552/1 -> cfblk3/1
  cyemi_553/1 -> cfblk4/1
  cfblk22/1 -> cyemi_553/1
  cyemi_554/1 -> cfblk4/2
  cyemi_555/1 -> cfblk8/1(cfblk1)
  cfblk14/1(cfblk2) -> cyemi_555/1
  cyemi_556/1 -> cfblk8/2(cfblk12)
  cyemi_557/1 -> cfblk8/3(cfblk13)
  cyemi_569/1 -> cfblk9/1(cfblk1)
  cyemi_570/1 -> cfblk9/2(cfblk6)
  cfblk3/1 -> cyemi_570/1

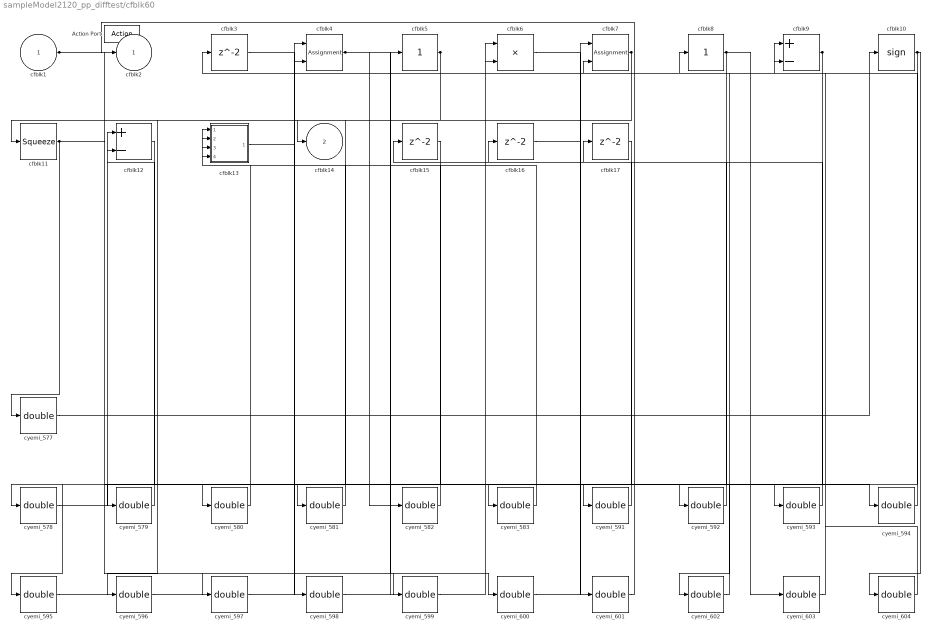
== system sampleModel2120_pp_difftest/cfblk60 ==
  cfblk1 : Inport
  Action Port : ActionPort  ActionPortLabel=if(u1 >= 0)
  cfblk10 : Signum
  cfblk11 : Squeeze
  cfblk12 : Sum  Inputs=+-  OutDataTypeStr=double
  cfblk13 : Subsystem
  cfblk{3,15..17} (4 alike) : Delay
  cfblk4 : Assignment  DiagnosticForDimensions=Warning  IndexOptions=Index vector (dialog)  Indices=1  OutputSizes=1
  cfblk5 : simulink/Math Operations/Slider Gain  gain=1  low=0  high=2
  cfblk6 : Product  OutDataTypeStr=double
  cfblk7 : Assignment  DiagnosticForDimensions=Warning  IndexOptions=Index vector (dialog)  Indices=1  OutputSizes=1
  cfblk8 : simulink/Math Operations/Slider Gain  gain=1  low=0  high=2
  cfblk9 : Sum  Inputs=+-  OutDataTypeStr=double
  cyemi_{577..583,591..604} (21 alike) : DataTypeConversion  OutDataTypeStr=double
  cfblk2 : Outport
  cfblk14 : Outport  Port=2
  wires:
  cfblk7/1 -> cfblk11/1, cyemi_581/1
  cfblk11/1 -> cyemi_577/1, cyemi_583/1, cyemi_599/1
  cfblk10/1 -> cyemi_602/1, cyemi_604/1
  cfblk5/1 -> cfblk14/1, cyemi_579/1
  cfblk4/1 -> cyemi_582/1, cyemi_600/1
  cfblk9/1 -> cfblk2/1, cyemi_591/1
  cfblk1/1 -> cyemi_580/1, cyemi_597/1
  cfblk8/1 -> cyemi_592/1, cyemi_603/1
  cyemi_577/1 -> cfblk10/1
  cyemi_578/1 -> cfblk12/1
  cfblk17/1 -> cyemi_578/1
  cyemi_579/1 -> cfblk12/2
  cyemi_580/1 -> cfblk13/1(cfblk1)
  cyemi_581/1 -> cfblk13/2(cfblk7)
  cyemi_582/1 -> cfblk13/3(cfblk8)
  cyemi_583/1 -> cfblk13/4(cfblk9)
  cyemi_591/1 -> cfblk15/1
  cyemi_592/1 -> cfblk16/1
  cyemi_593/1 -> cfblk17/1
  cfblk3/1 -> cyemi_593/1
  cyemi_594/1 -> cfblk3/1
  cfblk6/1 -> cyemi_594/1
  cyemi_595/1 -> cfblk4/1
  cfblk12/1 -> cyemi_595/1
  cyemi_596/1 -> cfblk4/2
  cfblk15/1 -> cyemi_596/1
  cyemi_597/1 -> cfblk5/1
  cyemi_598/1 -> cfblk6/1
  cfblk13/1(cfblk2) -> cyemi_598/1
  cyemi_599/1 -> cfblk6/2
  cyemi_600/1 -> cfblk7/1
  cyemi_601/1 -> cfblk7/2
  cfblk16/1 -> cyemi_601/1
  cyemi_602/1 -> cfblk8/1
  cyemi_603/1 -> cfblk9/1
  cyemi_604/1 -> cfblk9/2

== system sampleModel2120_pp_difftest/cfblk61 ==
  cfblk1 : Inport
  cfblk12 : Inport  Port=2
  cfblk13 : Inport  Port=3
  Action Port : ActionPort  ActionPortLabel=else
  cfblk10 : Subsystem
  cfblk11 : Subsystem
  cfblk15 : Delay
  cfblk3 : Delay  DelayLengthSource=Input port
      settings: InputPortMap=u0,p1
  cfblk4 : Delay
  cfblk5 : simulink/Math Operations/Slider Gain  gain=1  low=0  high=2
  cfblk6 : Sqrt  OutDataTypeStr=double  SaturateOnIntegerOverflow=on
  cfblk7 : Constant  Value=[999796448.984934]  OutDataTypeStr=double  SampleTime=1
  cfblk8 : Constant  Value=[-825546271.964894]  OutDataTypeStr=double  SampleTime=1
  cfblk9 : Constant  Value=[-268532313.679241]  OutDataTypeStr=double  SampleTime=1
  cyemi_{608..611,617,625..630} (11 alike) : DataTypeConversion  OutDataTypeStr=double
  cfblk2 : Outport
  cfblk14 : Outport  Port=2
  wires:
  cfblk6/1 -> cfblk2/1
  cfblk7/1 -> cfblk14/1
  cyemi_608/1 -> cfblk10/1(cfblk1)
  cfblk11/2(cfblk7) -> cyemi_608/1
  cyemi_609/1 -> cfblk10/2(cfblk8)
  cfblk12/1 -> cyemi_609/1
  cyemi_610/1 -> cfblk10/3(cfblk9)
  cfblk13/1 -> cyemi_610/1
  cyemi_611/1 -> cfblk10/4(cfblk10)
  cfblk8/1 -> cyemi_611/1
  cyemi_617/1 -> cfblk11/1(cfblk1)
  cfblk1/1 -> cyemi_617/1
  cyemi_625/1 -> cfblk15/1
  cfblk5/1 -> cyemi_625/1
  cyemi_626/1 -> cfblk3/1
  cfblk15/1 -> cyemi_626/1
  cyemi_627/1 -> cfblk3/2
  cfblk11/1(cfblk2) -> cyemi_627/1
  cyemi_628/1 -> cfblk4/1
  cfblk3/1 -> cyemi_628/1
  cyemi_629/1 -> cfblk5/1
  cfblk4/1 -> cyemi_629/1
  cyemi_630/1 -> cfblk6/1
  cfblk9/1 -> cyemi_630/1

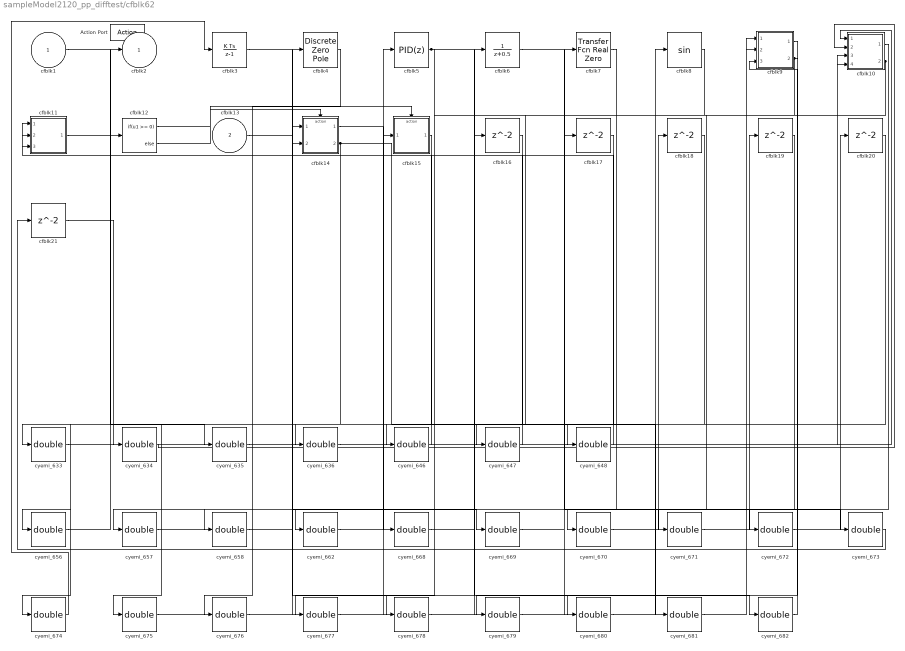
== system sampleModel2120_pp_difftest/cfblk62 ==
  cfblk1 : Inport
  cfblk13 : Inport  Port=2
  Action Port : ActionPort  ActionPortLabel=if(u1 >= 0)
  cfblk10 : Subsystem
  cfblk11 : Subsystem
  cfblk12 : If  IfExpression=u1 >= 0  SampleTime=1
  cfblk14 : Subsystem  TreatAsAtomicUnit=on
  cfblk15 : Subsystem  TreatAsAtomicUnit=on
  cfblk{16..21} (6 alike) : Delay
  cfblk3 : DiscreteIntegrator  SampleTime=-1  OutDataTypeStr=double  ICPrevOutput=DiscIntNeverNeededParam  ICPrevScaledInput=DiscIntNeverNeededParam
  cfblk4 : DiscreteZeroPole  Poles=[0 0.5]  Gain=1  SampleTime=-1
  cfblk5 : pid_lib/PID Controller  Controller=PID  Form=Parallel  TimeDomain=Discrete-time  UseExternalTs=off  SampleTime=-1  IntegratorMethod=Forward Euler  FilterMethod=Forward Euler  ControllerParametersSource=internal  P=1  I=1  D=0  UseFilter=on  N=100  TunerSelectOption=Transfer Function Based (PID Tuner App)  InitialConditionSource=internal  InitialConditionForIntegrator=0  InitialConditionForFilter=0  DifferentiatorICPrevScaledInput=0  ExternalReset=none  TrackingMode=off  Kt=1  LimitOutput=off  SatLimitsSource=internal  UpperSaturationLimit=inf  LowerSaturationLimit=-inf  LinearizeAsGain=off  AntiWindupMode=none  Kb=1  POutMin=[]  POutMax=[]  IOutMin=[]  IOutMax=[]  DOutMin=[]  DOutMax=[]  NOutMin=[]  NOutMax=[]  SumOutMin=[]  SumOutMax=[]  SaturationOutMin=[]  SaturationOutMax=[]  PParamMin=[]  PParamMax=[]  IParamMin=[]  IParamMax=[]  DParamMin=[]  DParamMax=[]  NParamMin=[]  NParamMax=[]  KbParamMin=[]  KbParamMax=[]  KtParamMin=[]  KtParamMax=[]  KbOutMin=[]  KbOutMax=[]  KtOutMin=[]  KtOutMax=[]  IntegratorOutMin=[]  IntegratorOutMax=[]  FilterOutMin=[]  FilterOutMax=[]  SumI1OutMin=[]  SumI1OutMax=[]  SumI2OutMin=[]  SumI2OutMax=[]  SumI3OutMin=[]  SumI3OutMax=[]  SumI4OutMin=[]  SumI4OutMax=[]  SumDOutMin=[]  SumDOutMax=[]  DifferentiatorOutMin=[]  DifferentiatorOutMax=[]  FilterDiffOutCoefMin=[]  FilterDiffOutCoefMax=[]  ReciprocalOutMin=[]  ReciprocalOutMax=[]  SumDenOutMin=[]  SumDenOutMax=[]  SumNumOutMin=[]  SumNumOutMax=[]  DivideOutMin=[]  DivideOutMax=[]  UdiffTsProdOutMin=[]  UdiffTsProdOutMax=[]  NTsProdOutMin=[]  NTsProdOutMax=[]  UintegralTsProdOutMin=[]  UintegralTsProdOutMax=[]  UngainTsProdOutMin=[]  UngainTsProdOutMax=[]  IntegratorContinuousStateAttributes=''  IntegratorStateMustResolveToSignalObject=off  IntegratorRTWStateStorageClass=Auto  FilterContinuousStateAttributes=''  FilterStateMustResolveToSignalObject=off  FilterRTWStateStorageClass=Auto  ParallelPVariant=InternalParameters  IdealPVariant=Disabled  IVariant=InternalParameters  DVariant=InternalParameters  IntegratorVariant=Discrete  SatVariant=Disabled  AWVariant=Passthrough  PCopyVariant=Disabled  TRVariant=Disabled  FdbkBlocksVariant=Forward  IdealPFdbkVariant=Disabled  SatFdbkVariant=Disabled  DerivativeFilterVariant=ForwardEulerFilter  NVariant=InternalParameters  NCopyVariant=Disabled  FilterICVariant=InternalICsFilter  IntegratorICVariant=InternalICs  ExternalResetVariant=Disabled  TRSumVariant=Passthrough  SumFdbkVariant=Disabled  SumVariant=Sum_PID  TsampFilterVariant=InternalTs  TsampNgainVariant=Passthrough  TsampIntegralVariant=Passthrough  ExternalSaturationOutDataTypeStr=Inherit: Same as second input
  cfblk6 : DiscreteTransferFcn
  cfblk7 : simulink/Discrete/Transfer Fcn Real Zero  ZeroZ=0.75  ICPrevInput=0.0  DoSatur=off
      settings: SourceProductBaseCode=SL
  cfblk8 : Trigonometry
  cfblk9 : Subsystem
  cyemi_{633..636,646..648,656..658,662,668..682} (26 alike) : DataTypeConversion  OutDataTypeStr=double
  cfblk2 : Outport
  wires:
  cfblk5/1 -> cyemi_678/1, cyemi_682/1
  cfblk14/2(cfblk8) -> cyemi_675/1, cyemi_681/1
  cfblk11/1(cfblk2) -> cfblk2/1
  cfblk9/2(cfblk12) -> cyemi_648/1, cyemi_671/1, cyemi_672/1
  cfblk10/2(cfblk14) -> cyemi_647/1, cyemi_677/1
  cfblk12/1 -> cfblk14/Action
  cfblk12/2 -> cfblk15/Action
  cyemi_633/1 -> cfblk10/1(cfblk1)
  cfblk18/1 -> cyemi_633/1
  cyemi_634/1 -> cfblk10/2(cfblk11)
  cfblk21/1 -> cyemi_634/1
  cyemi_635/1 -> cfblk10/3(cfblk12)
  cfblk1/1 -> cyemi_635/1
  cyemi_636/1 -> cfblk10/4(cfblk13)
  cfblk20/1 -> cyemi_636/1
  cyemi_646/1 -> cfblk11/1(cfblk1)
  cfblk8/1 -> cyemi_646/1
  cyemi_647/1 -> cfblk11/2(cfblk7)
  cyemi_648/1 -> cfblk11/3(cfblk8)
  cyemi_656/1 -> cfblk12/1
  cfblk16/1 -> cyemi_656/1
  cyemi_657/1 -> cfblk14/1(cfblk1)
  cfblk10/1(cfblk2) -> cyemi_657/1
  cyemi_658/1 -> cfblk14/2(cfblk7)
  cfblk17/1 -> cyemi_658/1
  cyemi_662/1 -> cfblk15/1(cfblk1)
  cfblk19/1 -> cyemi_662/1
  cyemi_668/1 -> cfblk16/1
  cfblk14/1(cfblk2) -> cyemi_668/1
  cyemi_669/1 -> cfblk17/1
  cfblk3/1 -> cyemi_669/1
  cyemi_670/1 -> cfblk18/1
  cfblk7/1 -> cyemi_670/1
  cyemi_671/1 -> cfblk19/1
  cyemi_672/1 -> cfblk20/1
  cyemi_673/1 -> cfblk21/1
  cfblk6/1 -> cyemi_673/1
  cyemi_674/1 -> cfblk3/1
  cfblk15/1(cfblk2) -> cyemi_674/1
  cyemi_675/1 -> cfblk4/1
  cyemi_676/1 -> cfblk5/1
  cfblk4/1 -> cyemi_676/1
  cyemi_677/1 -> cfblk6/1
  cyemi_678/1 -> cfblk7/1
  cyemi_679/1 -> cfblk8/1
  cfblk9/1(cfblk2) -> cyemi_679/1
  cyemi_680/1 -> cfblk9/1(cfblk1)
  cfblk13/1 -> cyemi_680/1
  cyemi_681/1 -> cfblk9/2(cfblk10)
  cyemi_682/1 -> cfblk9/3(cfblk11)

== system sampleModel2120_pp_difftest/cfblk63 ==
  cfblk1 : Inport
  Action Port : ActionPort  ActionPortLabel=else
  cfblk10 : Delay
  cfblk11 : DataTypeConversion  OutDataTypeStr=uint32
  cfblk12 : DataTypeConversion  OutDataTypeStr=double
  cfblk3 : DiscreteFilter
  cfblk4 : Delay  DelayLengthSource=Input port
      settings: InputPortMap=u0,p1
  cfblk5 : Sin  TimeSource=Use external signal  SampleTime=0
  cfblk6 : PermuteDimensions
  cfblk7 : Subsystem
  cfblk9 : Delay
  cyemi_{696..697,699..700,702,704,706} (7 alike) : DataTypeConversion  OutDataTypeStr=double
  cyemi_{698,701,703,705,714} (5 alike) : DataTypeConversion  OutDataTypeStr=uint32
  cfblk2 : Outport
  cfblk8 : Outport  Port=2
  wires:
  cfblk5/1 -> cfblk8/1
  cfblk1/1 -> cyemi_702/1, cyemi_706/1
  cfblk6/1 -> cyemi_701/1, cyemi_714/1
  cfblk7/2(cfblk11) -> cfblk2/1
  cyemi_696/1 -> cfblk10/1
  cfblk4/1 -> cyemi_696/1
  cyemi_697/1 -> cfblk11/1
  cfblk3/1 -> cyemi_697/1
  cyemi_698/1 -> cfblk12/1
  cfblk7/1(cfblk2) -> cyemi_698/1
  cyemi_699/1 -> cfblk3/1
  cfblk12/1 -> cyemi_699/1
  cyemi_700/1 -> cfblk4/1
  cfblk7/3(cfblk12) -> cyemi_700/1
  cyemi_701/1 -> cfblk4/2
  cyemi_702/1 -> cfblk5/1
  cyemi_703/1 -> cfblk6/1
  cfblk11/1 -> cyemi_703/1
  cyemi_704/1 -> cfblk7/1(cfblk1)
  cfblk10/1 -> cyemi_704/1
  cyemi_705/1 -> cfblk7/2(cfblk9)
  cfblk9/1 -> cyemi_705/1
  cyemi_706/1 -> cfblk7/3(cfblk10)
  cyemi_714/1 -> cfblk9/1

== system sampleModel2120_pp_difftest/cfblk45/cfblk10 ==
  cfblk1 : Inport
  cfblk10 : Sum  Inputs=+  OutDataTypeStr=double
  cfblk11 : Bias  Bias=[143732452.396222]
  cfblk3 : DiscreteFir  SampleTime=1
  cfblk4 : simulink/Discrete/Transfer Fcn Real Zero  ZeroZ=0.75  ICPrevInput=0.0  DoSatur=off
      settings: SourceProductBaseCode=SL
  cfblk5 : simulink/Discrete/Transfer Fcn First Order  PoleZ=0.95  ICPrevOutput=0.0  DoSatur=off
  cfblk6 : Delay  DelayLengthSource=Input port  SampleTime=1
      settings: InputPortMap=u0,p1
  cfblk7 : Bias  Bias=[415695908.441253]
  cfblk8 : simulink/Math Operations/Slider Gain  gain=1  low=0  high=2
  cfblk9 : Rounding
  cyemi_{24..33} (10 alike) : DataTypeConversion  OutDataTypeStr=double
  cfblk2 : Outport
  wires:
  cfblk9/1 -> cfblk2/1
  cfblk11/1 -> cyemi_26/1, cyemi_30/1
  cyemi_24/1 -> cfblk10/1
  cfblk5/1 -> cyemi_24/1
  cyemi_25/1 -> cfblk11/1
  cfblk8/1 -> cyemi_25/1
  cyemi_26/1 -> cfblk3/1
  cyemi_27/1 -> cfblk4/1
  cfblk3/1 -> cyemi_27/1
  cyemi_28/1 -> cfblk5/1
  cfblk4/1 -> cyemi_28/1
  cyemi_29/1 -> cfblk6/1
  cfblk10/1 -> cyemi_29/1
  cyemi_30/1 -> cfblk6/2
  cyemi_31/1 -> cfblk7/1
  cfblk1/1 -> cyemi_31/1
  cyemi_32/1 -> cfblk8/1
  cfblk7/1 -> cyemi_32/1
  cyemi_33/1 -> cfblk9/1
  cfblk6/1 -> cyemi_33/1

== system sampleModel2120_pp_difftest/cfblk45/cfblk11 ==
  cfblk1 : Inport
  cfblk6 : Inport  Port=2
  cfblk7 : Inport  Port=3
  cfblk8 : Inport  Port=4
  cfblk9 : Inport  Port=5
  cfblk3 : Sum  Inputs=-+  OutDataTypeStr=double
  cfblk4 : Constant  Value=[-156405987.882864]  OutDataTypeStr=double  SampleTime=1
  cfblk5 : Constant  Value=[-751982074.552397]  OutDataTypeStr=double  SampleTime=1
  cyemi_39 : DataTypeConversion  OutDataTypeStr=double
  cyemi_40 : DataTypeConversion  OutDataTypeStr=double
  cfblk2 : Outport
  cfblk10 : Outport  Port=2
  wires:
  cfblk4/1 -> cfblk10/1
  cfblk5/1 -> cfblk2/1
  cyemi_39/1 -> cfblk3/1
  cfblk8/1 -> cyemi_39/1
  cyemi_40/1 -> cfblk3/2
  cfblk7/1 -> cyemi_40/1

== system sampleModel2120_pp_difftest/cfblk45/cfblk12 ==
  cfblk1 : Inport
  cfblk11 : Inport  Port=2
  cfblk10 : Constant  Value=[257671330.793710]  OutDataTypeStr=double  SampleTime=1
  cfblk12 : Delay  SampleTime=1
  cfblk3 : simulink/Discrete/Transfer Fcn First Order  PoleZ=0.95  ICPrevOutput=0.0  DoSatur=off
  cfblk4 : Delay  ShowEnablePort=on  SampleTime=1
      settings: InputPortMap=u0,e6
  cfblk5 : DiscreteFilter  SampleTime=1
  cfblk6 : Product  OutDataTypeStr=double
  cfblk7 : Sum  Inputs=--  OutDataTypeStr=double
  cfblk8 : Sum  OutDataTypeStr=double
  cfblk9 : Constant  Value=[-533370526.019482]  OutDataTypeStr=double  SampleTime=1
  cyemi_{43..53} (11 alike) : DataTypeConversion  OutDataTypeStr=double
  cfblk2 : Outport
  wires:
  cfblk5/1 -> cfblk2/1
  cfblk1/1 -> cyemi_46/1, cyemi_50/1
  cyemi_43/1 -> cfblk12/1
  cfblk4/1 -> cyemi_43/1
  cyemi_44/1 -> cfblk3/1
  cfblk10/1 -> cyemi_44/1
  cyemi_45/1 -> cfblk4/1
  cfblk8/1 -> cyemi_45/1
  cyemi_46/1 -> cfblk4/2
  cyemi_47/1 -> cfblk5/1
  cfblk9/1 -> cyemi_47/1
  cyemi_48/1 -> cfblk6/1
  cfblk7/1 -> cyemi_48/1
  cyemi_49/1 -> cfblk6/2
  cfblk12/1 -> cyemi_49/1
  cyemi_50/1 -> cfblk7/1
  cyemi_51/1 -> cfblk7/2
  cfblk11/1 -> cyemi_51/1
  cyemi_52/1 -> cfblk8/1
  cfblk3/1 -> cyemi_52/1
  cyemi_53/1 -> cfblk8/2
  cfblk6/1 -> cyemi_53/1
